simulink model "OpenFAST_SFunc_NREL5MW_FF"  (R2022a)
settings: Solver=ode4  StartTime=0.0  StopTime=TMax  FixedStep=DT  MaxStep=DT  RelTol=1e-3  EnableMultiTasking=on
values from neighbouring files (symbols this model uses):
  Gd_Fwave = c2d(Sys{OperatingPoint}('omega_r','F_{hydro}'),Control.TimeStep,'tustin')    [ControlParams_NREL5MW.m]
  Gd_Mwave = c2d(Sys{OperatingPoint}('omega_r','M_{hydro}'),Control.TimeStep,'tustin')    [ControlParams_NREL5MW.m]
  InvGp = inv(Gp)    [ControlParams_NREL5MW.m]
  Kff_gain = 0.3    [InitCompDISCON.m]
undefined symbols (not defined in the file or in its folder): Control, OutList, strmatch
settings Model: Creator=bjonkman  LastModifiedBy=Amr Hegazy
settings SolverCC: AlgebraicLoopSolver=TrustRegion  MaxZcPerStep=1
settings DataIOCC: LimitDataPoints=on  SaveFormat=Array  SignalLoggingSaveFormat=ModelDataLogs  SaveOutput=off  SaveTime=off  ReturnWorkspaceOutputs=off  SignalLoggingName=sigsOut
settings OptimizationCC: ExpressionDepthLimit=2147483647  LifeSpan=inf
settings DebuggingCC: SaveWithParameterizedLinksMsg=none  UnderspecifiedInitializationDetection=Classic  MergeDetectMultiDrivingBlocksExec=none  SignalResolutionControl=TryResolveAllWithWarning  MultiTaskDSMMsg=warning  MultiTaskCondExecSysMsg=none  FcnCallInpInsideContextMsg=warning  UnconnectedInputMsg=warning  UnconnectedOutputMsg=warning  UnconnectedLineMsg=warning  StateNameClashWarn=warning  SFUnexpectedBacktrackingDiag=warning  SFNoUnconditionalDefaultTransitionDiag=warning  SFExecutionAtInitializationDiag=none  SFMachineParentedDataDiag=warning  ArithmeticOperatorsInVariantConditions=warning
settings HardwareCC: ProdBitPerPointer=32  ProdBitPerSizeT=32  ProdBitPerPtrDiffT=32  ProdLargestAtomicFloat=None  ProdIntDivRoundTo=Undefined  ProdEndianess=Unspecified  ProdWordSize=32  ProdHWDeviceType=32-bit Generic  TargetUnknown=on
settings ModelReferenceCC: PropagateSignalLabelsOutOfModel=off
settings SFSimCC: SimUseLocalCustomCode=off  CustomCodeUndefinedFunction=UseInterfaceOnly
settings RTWCC: RTWUseLocalCustomCode=off
settings CodeAppCC: StateflowObjectComments=on
settings GRTTargetCC: TargetLangStandard=C89/C90 (ANSI)  CombineOutputUpdateFcns=off  GRTInterface=on
settings ConfigComp: CovMetricSettings=dw  CovSaveCumulativeToWorkspaceVar=on  CovSaveSingleToWorkspaceVar=on  CovExternalEMLEnable=off

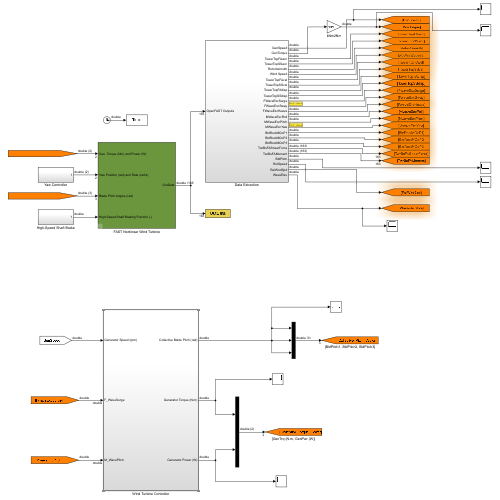
[thumbnail: Simulink's stored preview of the top-level diagram]
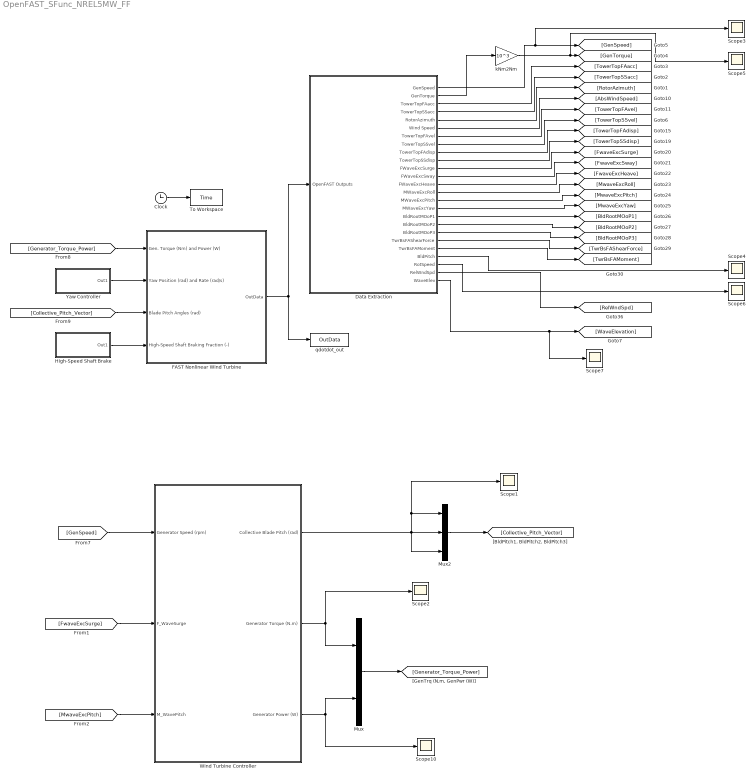
== system OpenFAST_SFunc_NREL5MW_FF ==
  Clock : Clock
  Data Extraction : Subsystem
  FAST Nonlinear Wind Turbine : Subsystem  mask(FAST Nonlinear Wind Turbine){}
      mask help: This block contains the FAST S-Function.
      mask init:
      | clear FAST_SFunc
  High-Speed Shaft Brake : Subsystem
  Mux : Mux  Inputs=2
  Mux2 : Mux  Inputs=3
  Scope{1..7,10} (8 alike) : Scope
  To Workspace : ToWorkspace  VariableName=Time  SampleTime=-1
  Wind Turbine Controller : Subsystem
  Yaw Controller : Subsystem
  kNm2Nm : Gain  Gain=10^3
  qdotdot_out : ToWorkspace  VariableName=OutData  SampleTime=-1
  wires:
  Clock/1 -> To Workspace/1
  FAST Nonlinear Wind Turbine/1(OutData) -> Data Extraction/1(OpenFAST Outputs), qdotdot_out/1
  Yaw Controller/1(Out1) -> FAST Nonlinear Wind Turbine/2(Yaw Position (rad) and Rate (rad/s))
  High-Speed Shaft Brake/1(Out1) -> FAST Nonlinear Wind Turbine/4(High-Speed Shaft Braking Fraction (-))
  Data Extraction/7(TowerTopFAvel) -> [TowerTopFAvel]
  Data Extraction/6(Wind Speed) -> [AbsWindSpeed]
  Data Extraction/4(TowerTopSSacc) -> [TowerTopSSacc]
  Data Extraction/3(TowerTopFAacc) -> [TowerTopFAacc]
  Data Extraction/2(GenTorque) -> kNm2Nm/1
  Data Extraction/8(TowerTopSSvel) -> [TowerTopSSvel]
  Data Extraction/9(TowerTopFAdisp) -> [TowerTopFAdisp]
  Data Extraction/10(TowerTopSSdisp) -> [TowerTopSSdisp]
  Data Extraction/11(FWaveExcSurge) -> [FwaveExcSurge]
  Data Extraction/12(FWaveExcSway) -> [FwaveExcSway]
  Data Extraction/13(FWaveExcHeave) -> [FwaveExcHeave]
  Data Extraction/14(MWaveExcRoll) -> [MwaveExcRoll]
  Data Extraction/15(MWaveExcPitch) -> [MwaveExcPitch]
  Data Extraction/16(MWaveExcYaw) -> [MwaveExcYaw]
  Data Extraction/17(BldRootMOoP1) -> [BldRootMOoP1]
  Data Extraction/18(BldRootMOoP2) -> [BldRootMOoP2]
  Data Extraction/19(BldRootMOoP3) -> [BldRootMOoP3]
  Data Extraction/21(TwrBsFAMoment) -> [TwrBsFAMoment]
  Data Extraction/20(TwrBsFAShearForce) -> [TwrBsFAShearForce]
  Data Extraction/1(GenSpeed) -> Scope3/1, [GenSpeed]
  kNm2Nm/1 -> Scope5/1, [GenTorque]
  Data Extraction/5(RotorAzimuth) -> [RotorAzimuth]
  Data Extraction/22(BldPitch) -> Scope4/1
  [Generator_Torque_Power] -> FAST Nonlinear Wind Turbine/1(Gen. Torque (Nm) and Power (W))
  [Collective_Pitch_Vector] -> FAST Nonlinear Wind Turbine/3(Blade Pitch Angles (rad))
  Data Extraction/23(RotSpeed) -> Scope6/1
  Mux2/1 -> [Collective_Pitch_Vector]
  Mux/1 -> [Generator_Torque_Power]
  [GenSpeed] -> Wind Turbine Controller/1(Generator Speed (rpm))
  Wind Turbine Controller/1(" Collective Blade Pitch (rad)") -> Scope1/1, Mux2/1, Mux2/3, Mux2/2
  Wind Turbine Controller/2(Generator Torque (N.m)) -> Scope2/1, Mux/1
  Wind Turbine Controller/3(Generator Power (W)) -> Mux/2, Scope10/1
  Data Extraction/24(RelWndSpd) -> [RelWndSpd]
  Data Extraction/25(WaveElev) -> Scope7/1, [WaveElevation]
  [FwaveExcSurge] -> Wind Turbine Controller/2(F_WaveSurge)
  [MwaveExcPitch] -> Wind Turbine Controller/3(M_WavePitch)

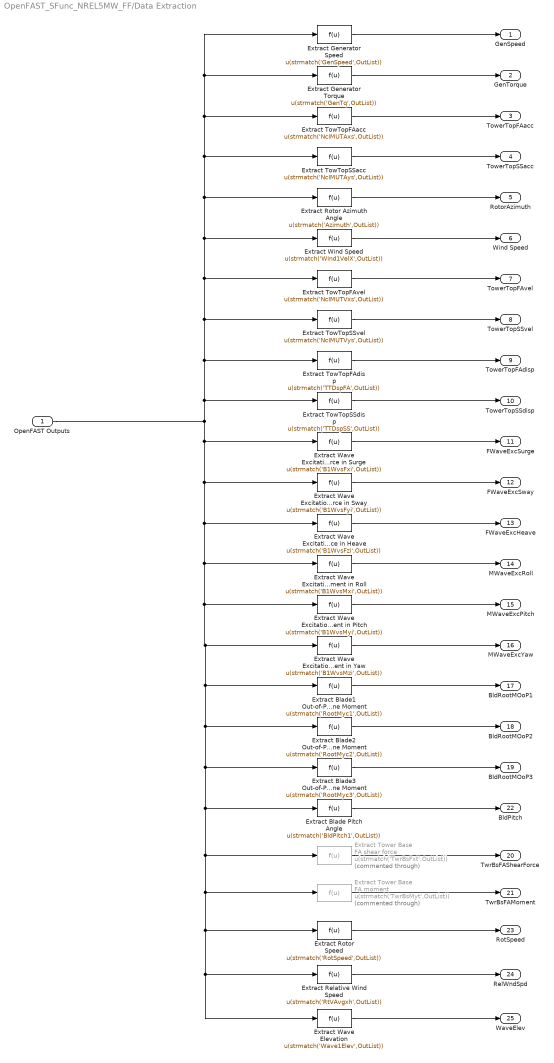
== system OpenFAST_SFunc_NREL5MW_FF/Data Extraction ==
  OpenFAST Outputs : Inport
  Extract Blade Pitch Angle : Fcn  Expr=u(strmatch('BldPitch1',OutList))
  Extract Blade1 Out-of-Plane Moment : Fcn  Expr=u(strmatch('RootMyc1',OutList))
  Extract Blade2 Out-of-Plane Moment : Fcn  Expr=u(strmatch('RootMyc2',OutList))
  Extract Blade3 Out-of-Plane Moment : Fcn  Expr=u(strmatch('RootMyc3',OutList))
  Extract Generator Speed : Fcn  Expr=u(strmatch('GenSpeed',OutList))
  Extract Generator Torque : Fcn  Expr=u(strmatch('GenTq',OutList))
  Extract Relative Wind Speed : Fcn  Expr=u(strmatch('RtVAvgxh',OutList))
  Extract Rotor Azimuth Angle : Fcn  Expr=u(strmatch('Azimuth',OutList))
  Extract Rotor Speed : Fcn  Expr=u(strmatch('RotSpeed',OutList))
  Extract TowTopFAacc : Fcn  Expr=u(strmatch('NcIMUTAxs',OutList))
  Extract TowTopFAdisp : Fcn  Expr=u(strmatch('TTDspFA',OutList))
  Extract TowTopFAvel : Fcn  Expr=u(strmatch('NcIMUTVxs',OutList))
  Extract TowTopSSacc : Fcn  Expr=u(strmatch('NcIMUTAys',OutList))
  Extract TowTopSSdisp : Fcn  Expr=u(strmatch('TTDspSS',OutList))
  Extract TowTopSSvel : Fcn  Expr=u(strmatch('NcIMUTVys',OutList))
  Extract Tower Base FA moment : Fcn  Commented=through  Expr=u(strmatch('TwrBsMyt',OutList))
  Extract Tower Base FA shear force : Fcn  Commented=through  Expr=u(strmatch('TwrBsFxt',OutList))
  Extract Wave Elevation : Fcn  Expr=u(strmatch('Wave1Elev',OutList))
  Extract Wave Excitation Force in Heave : Fcn  Expr=u(strmatch('B1WvsFzi',OutList))
  Extract Wave Excitation Force in Surge : Fcn  Expr=u(strmatch('B1WvsFxi',OutList))
  Extract Wave Excitation Force in Sway : Fcn  Expr=u(strmatch('B1WvsFyi',OutList))
  Extract Wave Excitation Moment in Pitch : Fcn  Expr=u(strmatch('B1WvsMyi',OutList))
  Extract Wave Excitation Moment in Roll : Fcn  Expr=u(strmatch('B1WvsMxi',OutList))
  Extract Wave Excitation Moment in Yaw : Fcn  Expr=u(strmatch('B1WvsMzi',OutList))
  Extract Wind Speed : Fcn  Expr=u(strmatch('Wind1VelX',OutList))
  GenSpeed : Outport
  GenTorque : Outport  Port=2
  TowerTopFAacc : Outport  Port=3
  TowerTopSSacc : Outport  Port=4
  RotorAzimuth : Outport  Port=5
  Wind Speed : Outport  Port=6
  TowerTopFAvel : Outport  Port=7
  TowerTopSSvel : Outport  Port=8
  TowerTopFAdisp : Outport  Port=9
  TowerTopSSdisp : Outport  Port=10
  FWaveExcSurge : Outport  Port=11
  FWaveExcSway : Outport  Port=12
  FWaveExcHeave : Outport  Port=13
  MWaveExcRoll : Outport  Port=14
  MWaveExcPitch : Outport  Port=15
  MWaveExcYaw : Outport  Port=16
  BldRootMOoP1 : Outport  Port=17
  BldRootMOoP2 : Outport  Port=18
  BldRootMOoP3 : Outport  Port=19
  TwrBsFAShearForce : Outport  Port=20
  TwrBsFAMoment : Outport  Port=21
  BldPitch : Outport  Port=22
  RotSpeed : Outport  Port=23
  RelWndSpd : Outport  Port=24
  WaveElev : Outport  Port=25
  wires:
  Extract Generator Speed/1 -> GenSpeed/1
  Extract Generator Torque/1 -> GenTorque/1
  Extract TowTopFAacc/1 -> TowerTopFAacc/1
  Extract TowTopSSacc/1 -> TowerTopSSacc/1
  Extract Rotor Azimuth Angle/1 -> RotorAzimuth/1
  Extract Wind Speed/1 -> Wind Speed/1
  Extract TowTopFAvel/1 -> TowerTopFAvel/1
  Extract TowTopSSvel/1 -> TowerTopSSvel/1
  Extract TowTopFAdisp/1 -> TowerTopFAdisp/1
  Extract TowTopSSdisp/1 -> TowerTopSSdisp/1
  Extract Wave Excitation Force in Surge/1 -> FWaveExcSurge/1
  Extract Wave Excitation Force in Sway/1 -> FWaveExcSway/1
  Extract Wave Excitation Force in Heave/1 -> FWaveExcHeave/1
  Extract Wave Excitation Moment in Roll/1 -> MWaveExcRoll/1
  Extract Wave Excitation Moment in Pitch/1 -> MWaveExcPitch/1
  Extract Wave Excitation Moment in Yaw/1 -> MWaveExcYaw/1
  Extract Blade1 Out-of-Plane Moment/1 -> BldRootMOoP1/1
  Extract Blade2 Out-of-Plane Moment/1 -> BldRootMOoP2/1
  Extract Blade3 Out-of-Plane Moment/1 -> BldRootMOoP3/1
  Extract Tower Base FA shear force/1 -> TwrBsFAShearForce/1
  Extract Tower Base FA moment/1 -> TwrBsFAMoment/1
  Extract Blade Pitch Angle/1 -> BldPitch/1
  Extract Rotor Speed/1 -> RotSpeed/1
  Extract Relative Wind Speed/1 -> RelWndSpd/1
  OpenFAST Outputs/1 -> Extract Blade Pitch Angle/1, Extract Wave Elevation/1, Extract Relative Wind Speed/1, Extract Rotor Speed/1, Extract Tower Base FA moment/1, Extract Tower Base FA shear force/1, Extract Blade3 Out-of-Plane Moment/1, Extract Blade2 Out-of-Plane Moment/1, Extract Blade1 Out-of-Plane Moment/1, Extract Wave Excitation Moment in Yaw/1, Extract Wave Excitation Moment in Pitch/1, Extract Wave Excitation Moment in Roll/1, Extract Wave Excitation Force in Heave/1, Extract Wave Excitation Force in Sway/1, Extract Wave Excitation Force in Surge/1, Extract Generator Speed/1, Extract Generator Torque/1, Extract TowTopFAacc/1, Extract TowTopSSacc/1, Extract Rotor Azimuth Angle/1, Extract Wind Speed/1, Extract TowTopFAvel/1, Extract TowTopSSvel/1, Extract TowTopFAdisp/1, Extract TowTopSSdisp/1
  Extract Wave Elevation/1 -> WaveElev/1

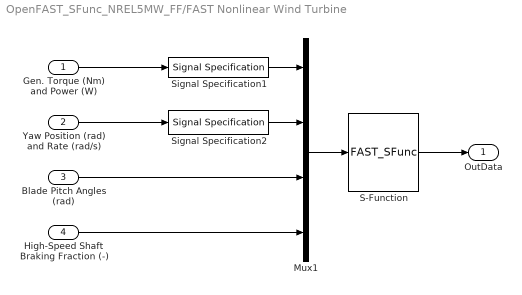
== system OpenFAST_SFunc_NREL5MW_FF/FAST Nonlinear Wind Turbine ==
  Gen. Torque (Nm) and Power (W) : Inport
  Yaw Position (rad) and Rate (rad/s) : Inport  Port=2
  Blade Pitch Angles (rad) : Inport  Port=3
  High-Speed Shaft Braking Fraction (-) : Inport  Port=4
  Mux1 : Mux
  S-Function : S-Function  FunctionName=FAST_SFunc  Parameters=FAST_InputFileName, TMax, 0  SFunctionDeploymentMode=off  EnableBusSupport=off
  Signal Specification1 : SignalSpecification  OutDataTypeStr=double  Dimensions=2
  Signal Specification2 : SignalSpecification  OutDataTypeStr=double  Dimensions=2
  OutData : Outport
  wires:
  Gen. Torque (Nm) and Power (W)/1 -> Signal Specification1/1
  S-Function/1 -> OutData/1
  Mux1/1 -> S-Function/1
  Blade Pitch Angles (rad)/1 -> Mux1/3
  Yaw Position (rad) and Rate (rad/s)/1 -> Signal Specification2/1
  Signal Specification1/1 -> Mux1/1
  Signal Specification2/1 -> Mux1/2
  High-Speed Shaft Braking Fraction (-)/1 -> Mux1/4

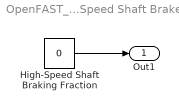
== system OpenFAST_SFunc_NREL5MW_FF/High-Speed Shaft Brake ==
  High-Speed Shaft Braking Fraction : Constant  Value=0
  Out1 : Outport
  wires:
  High-Speed Shaft Braking Fraction/1 -> Out1/1

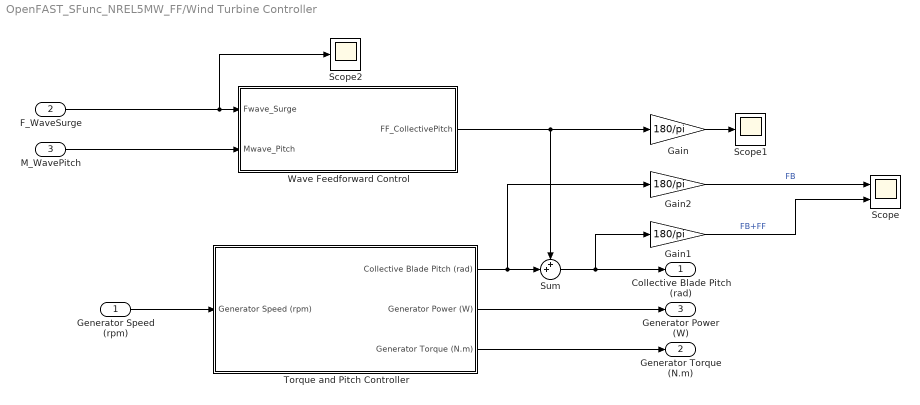
== system OpenFAST_SFunc_NREL5MW_FF/Wind Turbine Controller ==
  Generator Speed (rpm) : Inport
  F_WaveSurge : Inport  Port=2
  M_WavePitch : Inport  Port=3
  Gain : Gain  Gain=180/pi
  Gain1 : Gain  Gain=180/pi
  Gain2 : Gain  Gain=180/pi
  Scope : Scope  NumInputPorts=2
  Scope1 : Scope
  Scope2 : Scope
  Sum : Sum  Inputs=++|
  Torque and Pitch Controller : Subsystem
  Wave Feedforward Control : Subsystem
  " Collective Blade Pitch (rad)" : Outport
  Generator Torque (N.m) : Outport  Port=2
  Generator Power (W) : Outport  Port=3
  wires:
  Generator Speed (rpm)/1 -> Torque and Pitch Controller/1(Generator Speed (rpm))
  Torque and Pitch Controller/2(Generator Power (W)) -> Generator Power (W)/1
  Torque and Pitch Controller/3(Generator Torque (N.m)) -> Generator Torque (N.m)/1
  M_WavePitch/1 -> Wave Feedforward Control/2(Mwave_Pitch)
  F_WaveSurge/1 -> Scope2/1, Wave Feedforward Control/1(Fwave_Surge)
  Wave Feedforward Control/1(FF_CollectivePitch) -> Sum/1, Gain/1
  Torque and Pitch Controller/1(" Collective Blade Pitch (rad)") -> Gain2/1, Sum/2
  Sum/1 -> Gain1/1, " Collective Blade Pitch (rad)"/1
  Gain1/1 -> Scope/2  "FB+FF"
  Gain/1 -> Scope1/1
  Gain2/1 -> Scope/1  "FB"

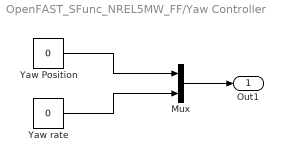
== system OpenFAST_SFunc_NREL5MW_FF/Yaw Controller ==
  Mux : Mux  Inputs=2
  Yaw Position : Constant  Value=0
  Yaw rate : Constant  Value=0
  Out1 : Outport
  wires:
  Mux/1 -> Out1/1
  Yaw Position/1 -> Mux/1
  Yaw rate/1 -> Mux/2

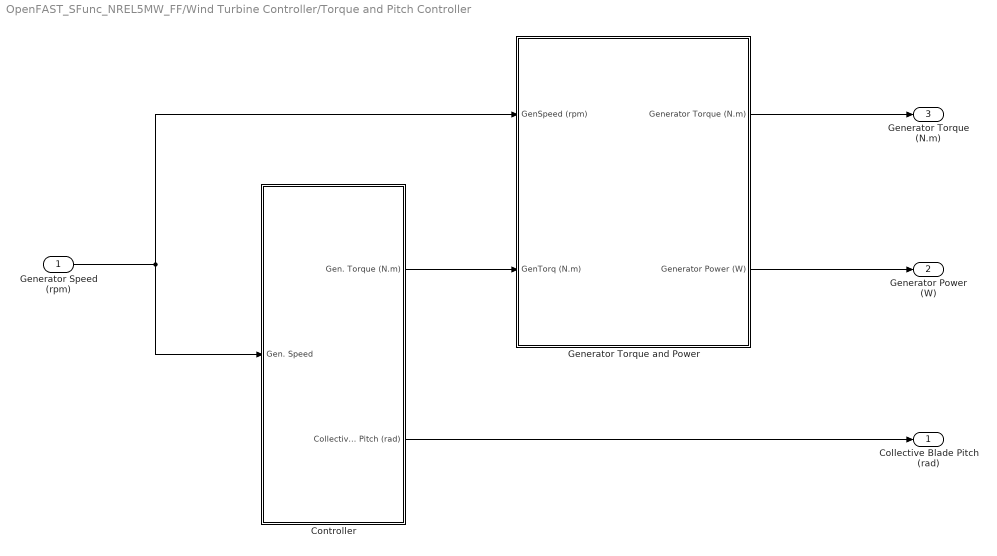
== system OpenFAST_SFunc_NREL5MW_FF/Wind Turbine Controller/Torque and Pitch Controller ==
  Generator Speed (rpm) : Inport
  Controller : Subsystem
  Generator Torque and Power : Subsystem
  " Collective Blade Pitch (rad)" : Outport
  Generator Power (W) : Outport  Port=2
  Generator Torque (N.m) : Outport  Port=3
  wires:
  Controller/1(Gen. Torque (N.m)) -> Generator Torque and Power/2(GenTorq (N.m))
  Generator Torque and Power/1(Generator Torque (N.m)) -> Generator Torque (N.m)/1
  Generator Torque and Power/2(Generator Power (W)) -> Generator Power (W)/1
  Generator Speed (rpm)/1 -> Generator Torque and Power/1(GenSpeed (rpm)), Controller/1(Gen. Speed)
  Controller/2(Collective Blade Pitch (rad)) -> " Collective Blade Pitch (rad)"/1

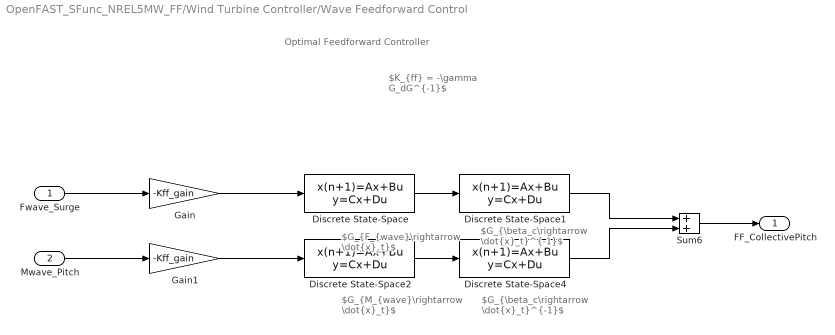
== system OpenFAST_SFunc_NREL5MW_FF/Wind Turbine Controller/Wave Feedforward Control ==
  note: $K_{ff} = -\gamma G_dG^{-1}$
  note: Optimal Feedforward Controller
  note: $G_{F_{wave}\rightarrow \dot{x}_t}$
  note: $G_{M_{wave}\rightarrow \dot{x}_t}$
  note: $G_{\beta_c\rightarrow \dot{x}_t}^{-1}$
  note: $G_{\beta_c\rightarrow \dot{x}_t}^{-1}$
  Fwave_Surge : Inport
  Mwave_Pitch : Inport  Port=2
  Discrete State-Space : DiscreteStateSpace  A=Gd_Fwave.A  B=Gd_Fwave.B  C=Gd_Fwave.C  D=Gd_Fwave.D  SampleTime=Control.TimeStep
  Discrete State-Space1 : DiscreteStateSpace  A=InvGp.A  B=InvGp.B  C=InvGp.C  D=InvGp.D  SampleTime=Control.TimeStep
  Discrete State-Space2 : DiscreteStateSpace  A=Gd_Mwave.A  B=Gd_Mwave.B  C=Gd_Mwave.C  D=Gd_Mwave.D  SampleTime=Control.TimeStep
  Discrete State-Space4 : DiscreteStateSpace  A=InvGp.A  B=InvGp.B  C=InvGp.C  D=InvGp.D  SampleTime=Control.TimeStep
  Gain : Gain  Gain=-Kff_gain
  Gain1 : Gain  Gain=-Kff_gain
  Sum6 : Sum
  FF_CollectivePitch : Outport
  wires:
  Fwave_Surge/1 -> Gain/1
  Gain/1 -> Discrete State-Space/1
  Discrete State-Space1/1 -> Sum6/1
  Gain1/1 -> Discrete State-Space2/1
  Mwave_Pitch/1 -> Gain1/1
  Sum6/1 -> FF_CollectivePitch/1
  Discrete State-Space2/1 -> Discrete State-Space4/1
  Discrete State-Space/1 -> Discrete State-Space1/1
  Discrete State-Space4/1 -> Sum6/2

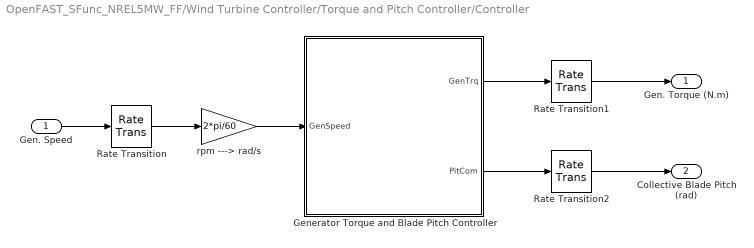
== system OpenFAST_SFunc_NREL5MW_FF/Wind Turbine Controller/Torque and Pitch Controller/Controller ==
  Gen. Speed : Inport
  Generator Torque and Blade Pitch Controller : MATLAB Function  TreatAsAtomicUnit=on
  Rate Transition : RateTransition
  Rate Transition1 : RateTransition
  Rate Transition2 : RateTransition
  rpm ---> rad/s : Gain  Gain=2*pi/60
  Gen. Torque (N.m) : Outport
  Collective Blade Pitch (rad) : Outport  Port=2
  wires:
  Gen. Speed/1 -> Rate Transition/1
  Rate Transition/1 -> rpm ---> rad/s/1
  rpm ---> rad/s/1 -> Generator Torque and Blade Pitch Controller/1(GenSpeed)
  Generator Torque and Blade Pitch Controller/1(GenTrq) -> Rate Transition1/1
  Rate Transition1/1 -> Gen. Torque (N.m)/1
  Generator Torque and Blade Pitch Controller/2(PitCom) -> Rate Transition2/1
  Rate Transition2/1 -> Collective Blade Pitch (rad)/1

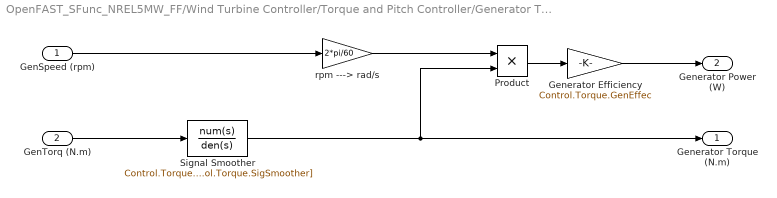
== system OpenFAST_SFunc_NREL5MW_FF/Wind Turbine Controller/Torque and Pitch Controller/Generator Torque and Power ==
  GenSpeed (rpm) : Inport
  GenTorq (N.m) : Inport  Port=2
  Generator Efficiency : Gain  Gain=Control.Torque.GenEffec
  Product : Product
  Signal Smoother : TransferFcn  Numerator=Control.Torque.SigSmoother  Denominator=[1 Control.Torque.SigSmoother]
  rpm ---> rad/s : Gain  Gain=2*pi/60
  Generator Torque (N.m) : Outport
  Generator Power (W) : Outport  Port=2
  wires:
  GenTorq (N.m)/1 -> Signal Smoother/1
  Generator Efficiency/1 -> Generator Power (W)/1
  Signal Smoother/1 -> Generator Torque (N.m)/1, Product/2
  Product/1 -> Generator Efficiency/1
  GenSpeed (rpm)/1 -> rpm ---> rad/s/1
  rpm ---> rad/s/1 -> Product/1

== matlab function OpenFAST_SFunc_NREL5MW_FF/Wind Turbine Controller/Torque and Pitch Controller/Controller/Generator Torque and Blade Pitch Controller ==
  data: GenTrq output; GenSpeed input; PitCom output; Control parameter
function [GenTrq, PitCom] = Controller(GenSpeed, Control)

%% Definition of the variables used in the script
% LPF_CornerFreq: Corner frequency (-3dB point) in the recursive, single-pole, low-pass filter, rad/s. -- chosen to be 1/4 the blade edgewise natural frequency ( 1/4 of approx. 1Hz = 0.25Hz = 1.570796rad/s)
% TimeStep      : Simulation time step (s)
% PC_DT         : Communication interval for pitch  controller, sec.
% PC_KI         : Integral gain for pitch controller at rated pitch (zero), (-).
% PC_KK         : Pitch angle where the the derivative of the aerodynamic power w.r.t. pitch has increased by a factor of two relative to the derivative at rated pitch (zero), rad.
% PC_KP         : Proportional gain for pitch controller at rated pitch (zero), sec.
% PC_MaxPit     : Maximum pitch setting in pitch controller, rad.
% PC_MaxRat     : Maximum pitch  rate (in absolute value) in pitch  controller, rad/s.
% PC_MinPit     : Minimum pitch setting in pitch controller, rad.
% PC_RefSpd     : Desired (reference) HSS speed for pitch controller, rad/s.
% PitCom        : Commanded pitch of each blade the last time the controller was called, rad.
% PitComI       : Integral term of command pitch, rad.
% PitComP       : Proportional term of command pitch, rad.
% PitComT       : Total command pitch based on the sum of the proportional and integral terms, rad.
% PitRate       : Pitch rates of each blade based on the current pitch angles and current pitch command, rad/s.
% SpdErr        : Current speed error, rad/s.
% TrqRate       : Torque rate based on the current and last torque commands, N-m/s.
% VS_CtInSp     : Transitional generator speed (HSS side) between regions 1 and 1 1/2, rad/s.
% VS_DT         : Communication interval for torque controller, sec.
% VS_MaxRat     : Maximum torque rate (in absolute value) in torque controller, N-m/s.
% VS_MaxTq      : Maximum generator torque in Region 3 (HSS side), N-m. -- chosen to be 10% above VS_RtTq = 43.09355kNm
% VS_Rgn2K      : Generator torque constant in Region 2 (HSS side), N-m/(rad/s)^2.
% VS_Rgn2Sp     : Transitional generator speed (HSS side) between regions 1 1/2 and 2, rad/s.
% VS_Rgn3MP     : Minimum pitch angle at which the torque is computed as if we are in region 3 regardless of the generator speed, rad. -- chosen to be 1.0 degree above PC_MinPit
% VS_RtGnSp     : Rated generator speed (HSS side), rad/s. -- chosen to be 99% of PC_RefSpd
% VS_RtPwr      : Rated generator generator power in Region 3, Watts. -- chosen to be 5MW divided by the electrical generator efficiency of 94.4%
% VS_Slope15    : Torque/speed slope of region 1 1/2 cut-in torque ramp , N-m/(rad/s).
% VS_Slope25    : Torque/speed slope of region 2 1/2 induction generator, N-m/(rad/s).
% VS_SlPc       : Rated generator slip percentage in Region 2 1/2, %.
% VS_SySp       : Synchronous speed of region 2 1/2 induction generator, rad/s.
% VS_TrGnSp     : Transitional generator speed (HSS side) between regions 2 and 2 1/2, rad/s.

% Note, each of the above variables is preceeded by the structure and the
% field where they are defined. That structure is called Control, and is
% composed of 4 field, namely, TimeStep, Filters, Torque and Pitch. 

%% Define the persistent variables in the function
persistent GenSpdFilt PitCommand GK SpdErrInt LastGenTorque 

%% Determine some torque control parameters not specified directly
VS_SySp       = Control.Torque.VS_RtGnSp/( 1.0 +  0.01*Control.Torque.VS_SlPc );                                                                         % Synchronous speed of region 2 1/2 induction generator, rad/s.
VS_Slope15    = (Control.Torque.VS_Rgn2K*Control.Torque.VS_Rgn2Sp*Control.Torque.VS_Rgn2Sp )/( Control.Torque.VS_Rgn2Sp - Control.Torque.VS_CtInSp );   % Torque/speed slope of region 1 1/2 cut-in torque ramp , N-m/(rad/s).
VS_Slope25    = ( Control.Torque.VS_RtPwr/Control.Pitch.PC_RefSpd           )/( Control.Torque.VS_RtGnSp - VS_SySp   );                                  % Torque/speed slope of region 2 1/2 induction generator , N-m/(rad/s).

if ( Control.Torque.VS_Rgn2K == 0.0 )
    VS_TrGnSp = VS_SySp;                                           % TRUE, if the torque in Region 2 is flat, and thus, the denominator in the ELSE condition is zero
else
    VS_TrGnSp = ( VS_Slope25 - sqrt( VS_Slope25*( VS_Slope25 - 4.0*Control.Torque.VS_Rgn2K*VS_SySp ) ) )/( 2.0*Control.Torque.VS_Rgn2K );
end

%% Initialize Saved Variables 
if isempty(GenSpdFilt)
    GenSpdFilt = GenSpeed;                                         % This will ensure that generator speed filter will use the initial value of the generator speed on the first pass                
    PitCommand = Control.Pitch.PC_MinPit;                          % This will ensure that the variable speed controller picks the correct control region and the pitch controller picks the correct gain on the first call
    GK         = 1.0/( 1.0 + PitCommand/Control.Pitch.PC_KK );     % This will ensure that the pitch angle is unchanged if the initial SpdErr is zero
    SpdErrInt  = PitCommand/( GK*Control.Pitch.PC_KI );            % This will ensure that the pitch angle is unchanged if the initial SpdErr is zero    
end

%% ============================= Filtering ============================= %%
% Filter the HSS (generator) speed measurement
% NOTE: This is a very simple recursive, single-pole, low-pass filter with exponential smoothing.
Alpha         = exp( -Control.TimeStep * Control.Filters.LPF_CornerFreq );

% Apply the Filter
GenSpeedF = ( 1.0 - Alpha )*GenSpeed + Alpha * GenSpdFilt;

% Update the persistent variable GenSpdFilt (This is to store the value of the presistent variable to be e used in the next time step)
GenSpdFilt = GenSpeedF;
     
%% =================== Variable-Speed Torque Control =================== %%
% Compute the generator torque, which depends on which region we are in:
if(GenSpeedF >= Control.Torque.VS_RtGnSp)||( PitCommand>= Control.Torque.VS_Rgn3MP )                   % We are in region 3 - power is constant
    GenTrq = Control.Torque.VS_RtPwr/Control.Pitch.PC_RefSpd;
elseif(GenSpeedF <= Control.Torque.VS_CtInSp)                                                          % We are in region 1 - torque is zero
    GenTrq = 0.0;
elseif(GenSpeedF <  Control.Torque.VS_Rgn2Sp)                                                          % We are in region 1 1/2 - linear ramp in torque from zero to optimal
    GenTrq = VS_Slope15*( GenSpeedF - Control.Torque.VS_CtInSp );
elseif(GenSpeedF <  VS_TrGnSp)                                                                         % We are in region 2 - optimal torque is proportional to the square of the generator speed
    GenTrq = Control.Torque.VS_Rgn2K*GenSpeedF*GenSpeedF;
else                                                                                                   % We are in region 2 1/2 - simple induction generator transition region
    GenTrq = VS_Slope25*( GenSpeedF - VS_SySp   );
end

% Saturate the commanded torque using the maximum torque limit:
GenTrq  = min( GenTrq, Control.Torque.VS_MaxTq  );                                                     % Saturate the command using the maximum torque limit

% Saturate the commanded torque using the torque rate limit:
if isempty(LastGenTorque)
    LastGenTorque = GenTrq;                                                                            % Initialize the value of LastGenTrq on the first pass only
end

TrqRate = ( GenTrq - LastGenTorque )/Control.TimeStep;                                                 % Torque rate (unsaturated)         
TrqRate = min( max( TrqRate, -Control.Torque.VS_MaxRat ), Control.Torque.VS_MaxRat );                  % Saturate the torque rate using its maximum absolute value
GenTrq  = LastGenTorque + TrqRate*Control.TimeStep;                                                    % Saturate the command using the torque rate limit

% Store the value of LastGenTorque for the next time step:
LastGenTorque = GenTrq;


%% =========================== Pitch Control =========================== %%

% Compute the gain scheduling correction factor based on the previously commanded pitch angle for blade 1:
GK = 1.0/( 1.0 + PitCommand/Control.Pitch.PC_KK );                    

% Compute the current speed error and its integral w.r.t. time;
% saturate the integral term using the pitch angle limits:
SpdErr    = GenSpdFilt - Control.Pitch.PC_RefSpd;                                                     % Current speed error        
IntSpdErr = SpdErrInt + SpdErr*Control.TimeStep;                                                      % Current integral of speed error w.r.t. time             
IntSpdErr = min( max( IntSpdErr, Control.Pitch.PC_MinPit/( GK*Control.Pitch.PC_KI ) ), Control.Pitch. PC_MaxPit/( GK*Control.Pitch.PC_KI ));    % Saturate the integral term using the pitch angle limits, converted to integral speed error limits

% Compute the pitch commands associated with the proportional and integral gains:
PitComP   = GK*Control.Pitch.PC_KP*SpdErr;                                                            % Proportional term          
PitComI   = GK*Control.Pitch.PC_KI*IntSpdErr;                                                         % Integral term (saturated) 

% Superimpose the individual commands to get the total pitch command;
%  saturate the overall command using the pitch angle limits:
PitComT   = PitComP + PitComI;                                                                        % Overall command (unsaturated)       
PitComT   = min( max( PitComT, Control.Pitch.PC_MinPit ), Control.Pitch.PC_MaxPit );                  % Saturate the overall command using the pitch angle limits

% Saturate the overall commanded pitch using the pitch rate limit:
% NOTE: Since the current pitch angle may be different for each blade
% (depending on the type of actuator implemented in the structural
% dynamics model), this pitch rate limit calculation and the 
% resulting overall pitch angle command may be different for each blade.
PitRate   = ( PitComT - PitCommand)/Control.TimeStep;                                                 % Pitch rate of the blades (unsaturated)           
PitRate   = min( max( PitRate, -Control.Pitch.PC_MaxRat ), Control.Pitch.PC_MaxRat );                 % Saturate the pitch rate of the blade using its maximum absolute value

PitCom    = PitCommand + PitRate*Control.TimeStep;                                                    % Saturate the overall command of the blade using the pitch rate limit           
PitCom    = min( max( PitCom, Control.Pitch.PC_MinPit ), Control.Pitch.PC_MaxPit );                   % Saturate the overall command using the pitch angle limits

% Store the persistent variables to be used in the next time step)
PitCommand = PitCom;
SpdErrInt = IntSpdErr;
